simulink model "nolinear_sina"  (Simulink 6.3)
settings: Solver=ode45  StartTime=0.0  StopTime=10.0  RelTol=1e-3
libraries: simulink x1
settings Model: LastModifiedBy=jiaosongming

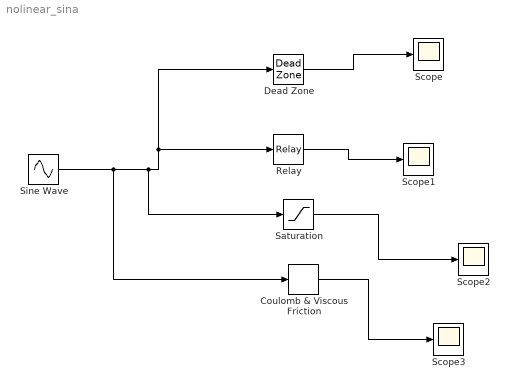
== system nolinear_sina ==
  Coulomb & Viscous Friction : simulink/Discontinuities/Coulomb & Viscous Friction  offset=[1 3 2 0]  gain=1
  Dead Zone : DeadZone  SaturateOnIntegerOverflow=on
  Relay : Relay
  Saturation : Saturate
  Scope{,1..3} (4 alike) : Scope
      Scope2 settings: SaveName=ScopeData2
      Scope3 settings: SaveName=ScopeData3
  Sine Wave : Sin  SampleTime=0
  wires:
  Sine Wave/1 -> Dead Zone/1, Relay/1, Saturation/1, Coulomb & Viscous Friction/1
  Dead Zone/1 -> Scope/1
  Relay/1 -> Scope1/1
  Saturation/1 -> Scope2/1
  Coulomb & Viscous Friction/1 -> Scope3/1
